simulink model "Quadrotor_Model_original"  (R2025b)
settings: Solver=ode45  StartTime=0.0  StopTime=15000  MaxStep=0.01  RelTol=1e-3  AbsTol=1e-4  EnableMultiTasking=on
values from neighbouring files (symbols this model uses):
  b = 0.07    [project_launch.m]
  g = 9.81    [project_launch.m]
  Jr = 1e-4    (= 0.0001)    [project_launch.m]
  k = 0.09    [project_launch.m]
  L = 0.225    [project_launch.m]
  m = 1.6    [project_launch.m]
libraries: slpidlib x5
settings Model: Creator=boyan  LastModifiedBy=neera
settings SolverCC: MaxConsecutiveMinStep=2  AlgebraicLoopSolver=TrustRegion
settings DataIOCC: LimitDataPoints=on  SaveFormat=Array  ReturnWorkspaceOutputs=off
settings OptimizationCC: LifeSpan=inf
settings DebuggingCC: SolverPrmCheckMsg=warning  UnconnectedInputMsg=warning  UnconnectedOutputMsg=warning  UnconnectedLineMsg=warning  SFUnexpectedBacktrackingDiag=warning  SFNoUnconditionalDefaultTransitionDiag=warning  SFExecutionAtInitializationDiag=none  ArithmeticOperatorsInVariantConditions=warning
settings HardwareCC: ProdBitPerPointer=32.0  ProdBitPerSizeT=32.0  ProdBitPerPtrDiffT=32.0  ProdLargestAtomicFloat=None  ProdIntDivRoundTo=Undefined  ProdEndianess=Unspecified  ProdWordSize=32.0  ProdHWDeviceType=32-bit Generic
settings ModelReferenceCC: EnableRefExpFcnMdlSchedulingChecks=on  PropagateSignalLabelsOutOfModel=off
settings SFSimCC: SimUseLocalCustomCode=off  CustomCodeUndefinedFunction=UseInterfaceOnly
settings RTWCC: RTWUseLocalCustomCode=off  GPUComputeCapability=3.5  DLArmComputeVersion=19.05
settings CodeAppCC: StateflowObjectComments=on
settings GRTTargetCC: TargetLangStandard=C89/C90 (ANSI)
settings ConfigComp: CovMetricSettings=dw  CovSaveCumulativeToWorkspaceVar=on  CovSaveSingleToWorkspaceVar=on  CovExternalEMLEnable=off  CovSFcnEnable=off

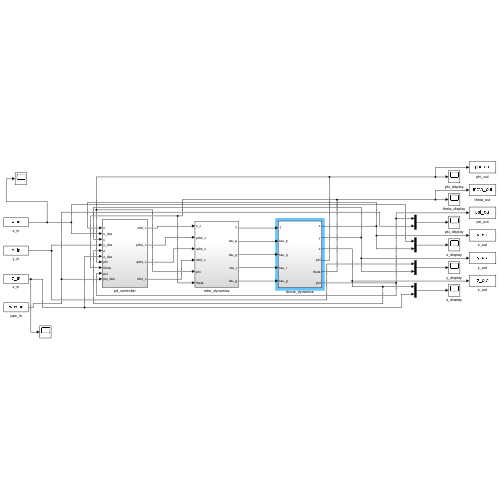
[thumbnail: Simulink's stored preview of the top-level diagram]
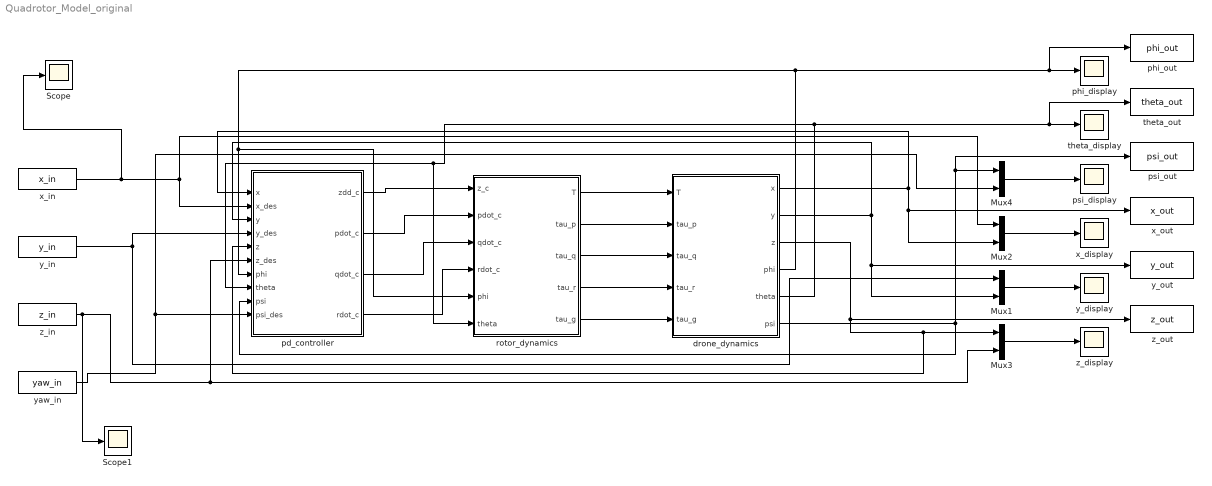
== system Quadrotor_Model_original ==
  Mux{1..4} (4 alike) : Mux  Inputs=2
  Scope : Scope
      settings: ActiveDisplayYMinimum=-3436.3102605592403  ActiveDisplayYMaximum=5145.090238480886  DataLoggingVariableName=ScopeData6
  Scope1 : Scope
      settings: ActiveDisplayYMinimum=-38.711321710722657  ActiveDisplayYMaximum=9.9150058205273481  DataLoggingVariableName=ScopeData7
  drone_dynamics : Subsystem
  pd_controller : Subsystem
  phi_display : Scope
      settings: ActiveDisplayYMinimum=-48.30659  ActiveDisplayYMaximum=31.01137
  phi_out : ToWorkspace  VariableName=phi_out  SaveFormat=Timeseries  SampleTime=-1
  psi_display : Scope
      settings: ActiveDisplayYMinimum=-104019.46579  ActiveDisplayYMaximum=26220.25866  DataLoggingVariableName=ScopeData2
  psi_out : ToWorkspace  VariableName=psi_out  SaveFormat=Timeseries  SampleTime=-1
  rotor_dynamics : Subsystem
  theta_display : Scope
      settings: ActiveDisplayYMinimum=-1.26378  ActiveDisplayYMaximum=0.84614  DataLoggingVariableName=ScopeData3
  theta_out : ToWorkspace  VariableName=theta_out  SaveFormat=Timeseries  SampleTime=-1
  x_display : Scope
      settings: ActiveDisplayYMinimum=-0.02581  ActiveDisplayYMaximum=0.17972  DataLoggingVariableName=ScopeData4
  x_in : FromWorkspace  VariableName=x_in
  x_out : ToWorkspace  VariableName=x_out  SaveFormat=Timeseries  SampleTime=-1
  y_display : Scope
      settings: ActiveDisplayYMinimum=98.09651  ActiveDisplayYMaximum=101.74643  DataLoggingVariableName=ScopeData5
  y_in : FromWorkspace  VariableName=y_in
  y_out : ToWorkspace  VariableName=y_out  SaveFormat=Timeseries  SampleTime=-1
  yaw_in : FromWorkspace  VariableName=yaw_in
  z_display : Scope
      settings: ActiveDisplayYMinimum=-47.57242  ActiveDisplayYMaximum=5.28582
  z_in : FromWorkspace  VariableName=z_in
  z_out : ToWorkspace  VariableName=z_out  SaveFormat=Timeseries  SampleTime=-1
  wires:
  rotor_dynamics/1(T) -> drone_dynamics/1(T)
  rotor_dynamics/2(tau_p) -> drone_dynamics/2(tau_p)
  pd_controller/1(zdd_c) -> rotor_dynamics/1(z_c)
  pd_controller/2(pdot_c) -> rotor_dynamics/2(pdot_c)
  z_in/1 -> pd_controller/6(z_des), Mux3/2, Scope1/1
  Mux1/1 -> y_display/1
  Mux2/1 -> x_display/1
  Mux4/1 -> psi_display/1
  Mux3/1 -> z_display/1
  drone_dynamics/6(psi) -> pd_controller/9(psi), psi_out/1, Mux4/1
  y_in/1 -> pd_controller/4(y_des), Mux1/1
  x_in/1 -> Scope/1, pd_controller/2(x_des), Mux2/1
  drone_dynamics/3(z) -> z_out/1, pd_controller/5(z), Mux3/1
  drone_dynamics/5(theta) -> theta_out/1, theta_display/1, pd_controller/8(theta), rotor_dynamics/6(theta)
  drone_dynamics/2(y) -> pd_controller/3(y), Mux1/2, y_out/1
  drone_dynamics/4(phi) -> phi_out/1, phi_display/1, pd_controller/7(phi), rotor_dynamics/5(phi)
  drone_dynamics/1(x) -> pd_controller/1(x), Mux2/2, x_out/1
  rotor_dynamics/5(tau_g) -> drone_dynamics/5(tau_g)
  rotor_dynamics/3(tau_q) -> drone_dynamics/3(tau_q)
  rotor_dynamics/4(tau_r) -> drone_dynamics/4(tau_r)
  yaw_in/1 -> pd_controller/10(psi_des), Mux4/2
  pd_controller/4(rdot_c) -> rotor_dynamics/4(rdot_c)
  pd_controller/3(qdot_c) -> rotor_dynamics/3(qdot_c)

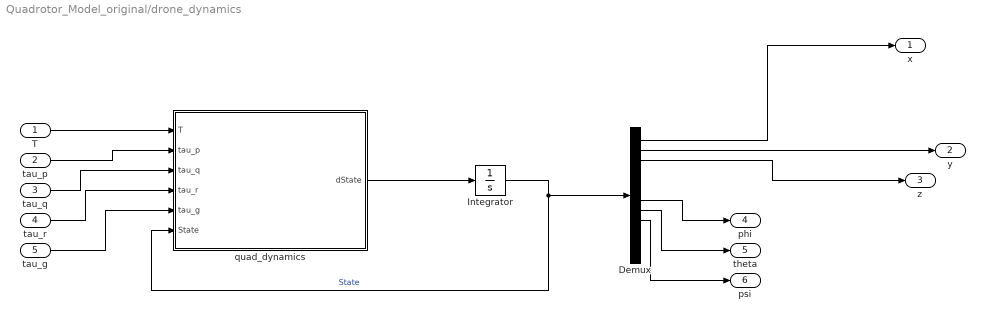
== system Quadrotor_Model_original/drone_dynamics ==
  T : Inport
  tau_p : Inport  Port=2
  tau_q : Inport  Port=3
  tau_r : Inport  Port=4
  tau_g : Inport  Port=5
  Demux : Demux  Outputs=12
  Integrator : Integrator  InitialCondition=[0; 0; 0; 0; 0; 0; 0; 0; 0; 0; 0; 0]
  quad_dynamics : MATLAB Function  TreatAsAtomicUnit=on
  x : Outport
  y : Outport  Port=2
  z : Outport  Port=3
  phi : Outport  Port=4
  theta : Outport  Port=5
  psi : Outport  Port=6
  wires:
  tau_p/1 -> quad_dynamics/2(tau_p)
  tau_q/1 -> quad_dynamics/3(tau_q)
  tau_r/1 -> quad_dynamics/4(tau_r)
  tau_g/1 -> quad_dynamics/5(tau_g)
  T/1 -> quad_dynamics/1(T)
  quad_dynamics/1(dState) -> Integrator/1
  Integrator/1 -> quad_dynamics/6(State), Demux/1  "State"
  Demux/7 -> phi/1
  Demux/8 -> theta/1
  Demux/9 -> psi/1
  Demux/1 -> x/1
  Demux/3 -> z/1
  Demux/2 -> y/1

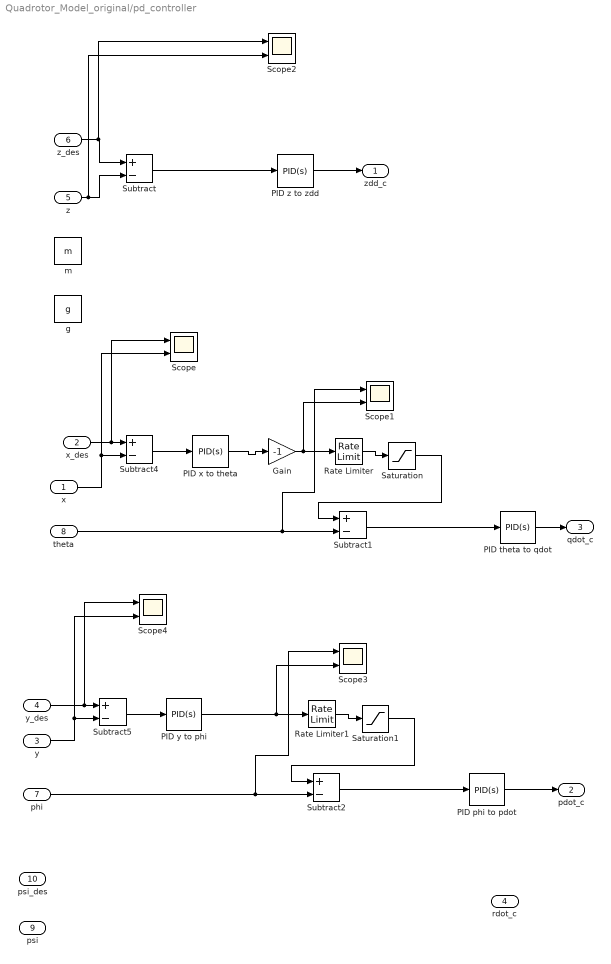
== system Quadrotor_Model_original/pd_controller ==
  x : Inport
  x_des : Inport  Port=2
  y : Inport  Port=3
  y_des : Inport  Port=4
  z : Inport  Port=5
  z_des : Inport  Port=6
  phi : Inport  Port=7
  theta : Inport  Port=8
  psi : Inport  Port=9
  psi_des : Inport  Port=10
  Gain : Gain  Gain=-1
  PID phi to pdot : slpidlib/PID Controller  Controller=PID  Form=Parallel  TimeDomain=Continuous-time  UseExternalTs=off  SampleTime=-1  IntegratorMethod=Forward Euler  FilterMethod=Forward Euler  ControllerParametersSource=internal  P=1  I=0  UseKiTs=off  D=0.5  UseExternalDerivativeSource=off  N=100  UseFilter=on  TunerSelectOption=Transfer Function Based (PID Tuner App)  InitialConditionSource=internal  InitialConditionForIntegrator=0  InitialConditionForFilter=0  DifferentiatorICPrevScaledInput=0  ExternalReset=none  TrackingMode=off  Kt=1  LimitOutput=off  SatLimitsSource=internal  UpperSaturationLimit=inf  LowerSaturationLimit=-inf  LinearizeAsGain=on  AntiWindupMode=none  Kb=1  LimitIntegrator=off  UpperIntegratorSaturationLimit=inf  LowerIntegratorSaturationLimit=-inf  POutMin=[]  POutMax=[]  IOutMin=[]  IOutMax=[]  DOutMin=[]  DOutMax=[]  NOutMin=[]  NOutMax=[]  SumOutMin=[]  SumOutMax=[]  SaturationOutMin=[]  SaturationOutMax=[]  PParamMin=[]  PParamMax=[]  IParamMin=[]  IParamMax=[]  DParamMin=[]  DParamMax=[]  NParamMin=[]  NParamMax=[]  KbParamMin=[]  KbParamMax=[]  KtParamMin=[]  KtParamMax=[]  KbOutMin=[]  KbOutMax=[]  KtOutMin=[]  KtOutMax=[]  IntegratorOutMin=[]  IntegratorOutMax=[]  FilterOutMin=[]  FilterOutMax=[]  SumI1OutMin=[]  SumI1OutMax=[]  SumI2OutMin=[]  SumI2OutMax=[]  SumI3OutMin=[]  SumI3OutMax=[]  SumI4OutMin=[]  SumI4OutMax=[]  SumDOutMin=[]  SumDOutMax=[]  DifferentiatorOutMin=[]  DifferentiatorOutMax=[]  FilterDiffOutCoefMin=[]  FilterDiffOutCoefMax=[]  ReciprocalOutMin=[]  ReciprocalOutMax=[]  SumDenOutMin=[]  SumDenOutMax=[]  SumNumOutMin=[]  SumNumOutMax=[]  DivideOutMin=[]  DivideOutMax=[]  UdiffTsProdOutMin=[]  UdiffTsProdOutMax=[]  NTsProdOutMin=[]  NTsProdOutMax=[]  UintegralTsProdOutMin=[]  UintegralTsProdOutMax=[]  UngainTsProdOutMin=[]  UngainTsProdOutMax=[]  ClampingZeroOutDataTypeStr=Inherit: Inherit via back propagation  ClampingZeroOutMin=[]  ClampingZeroOutMax=[]  FilterDenConstantOutDataTypeStr=Inherit: Inherit via back propagation  FilterDenConstantOutMin=[]  FilterDenConstantOutMax=[]  PCopyOutDataTypeStr=Inherit: Inherit via back propagation  PCopyOutMin=[]  PCopyOutMax=[]  NCopyOutDataTypeStr=Inherit: Inherit via back propagation  NCopyOutMin=[]  NCopyOutMax=[]  IntegratorContinuousStateAttributes=''  IntegratorStateMustResolveToSignalObject=off  IntegratorRTWStateStorageClass=Auto  FilterContinuousStateAttributes=''  FilterStateMustResolveToSignalObject=off  FilterRTWStateStorageClass=Auto  ParallelPVariant=InternalParameters  IdealPVariant=Disabled  IVariant=InternalParameters  DVariant=InternalParameters  IntegratorVariant=Continuous  SatVariant=Disabled  AWVariant=Passthrough  PCopyVariant=Disabled  TRVariant=Disabled  FdbkBlocksVariant=Forward  IdealPFdbkVariant=Disabled  SatFdbkVariant=Disabled  DerivativeFilterVariant=ContFilter  NVariant=InternalParameters  NCopyVariant=Disabled  FilterICVariant=InternalICsFilter  IntegratorICVariant=InternalICs  ExternalResetVariant=Disabled  TRSumVariant=Passthrough  SumFdbkVariant=Disabled  SumVariant=Sum_PID  TsampFilterVariant=InternalTs  TsampNgainVariant=Passthrough  TsampIntegralVariant=Disabled_SignalSpec  ExternalSaturationOutDataTypeStr=Inherit: Same as second input  DerivativeSourceVariant=ErrorSignal  PreIntVariant=InternalPreInt
  PID theta to qdot : slpidlib/PID Controller  Controller=PID  Form=Parallel  TimeDomain=Continuous-time  UseExternalTs=off  SampleTime=-1  IntegratorMethod=Forward Euler  FilterMethod=Forward Euler  ControllerParametersSource=internal  P=1  I=0  UseKiTs=off  D=0.5  UseExternalDerivativeSource=off  N=100  UseFilter=on  TunerSelectOption=Transfer Function Based (PID Tuner App)  InitialConditionSource=internal  InitialConditionForIntegrator=0  InitialConditionForFilter=0  DifferentiatorICPrevScaledInput=0  ExternalReset=none  TrackingMode=off  Kt=1  LimitOutput=off  SatLimitsSource=internal  UpperSaturationLimit=inf  LowerSaturationLimit=-inf  LinearizeAsGain=on  AntiWindupMode=none  Kb=1  LimitIntegrator=off  UpperIntegratorSaturationLimit=inf  LowerIntegratorSaturationLimit=-inf  POutMin=[]  POutMax=[]  IOutMin=[]  IOutMax=[]  DOutMin=[]  DOutMax=[]  NOutMin=[]  NOutMax=[]  SumOutMin=[]  SumOutMax=[]  SaturationOutMin=[]  SaturationOutMax=[]  PParamMin=[]  PParamMax=[]  IParamMin=[]  IParamMax=[]  DParamMin=[]  DParamMax=[]  NParamMin=[]  NParamMax=[]  KbParamMin=[]  KbParamMax=[]  KtParamMin=[]  KtParamMax=[]  KbOutMin=[]  KbOutMax=[]  KtOutMin=[]  KtOutMax=[]  IntegratorOutMin=[]  IntegratorOutMax=[]  FilterOutMin=[]  FilterOutMax=[]  SumI1OutMin=[]  SumI1OutMax=[]  SumI2OutMin=[]  SumI2OutMax=[]  SumI3OutMin=[]  SumI3OutMax=[]  SumI4OutMin=[]  SumI4OutMax=[]  SumDOutMin=[]  SumDOutMax=[]  DifferentiatorOutMin=[]  DifferentiatorOutMax=[]  FilterDiffOutCoefMin=[]  FilterDiffOutCoefMax=[]  ReciprocalOutMin=[]  ReciprocalOutMax=[]  SumDenOutMin=[]  SumDenOutMax=[]  SumNumOutMin=[]  SumNumOutMax=[]  DivideOutMin=[]  DivideOutMax=[]  UdiffTsProdOutMin=[]  UdiffTsProdOutMax=[]  NTsProdOutMin=[]  NTsProdOutMax=[]  UintegralTsProdOutMin=[]  UintegralTsProdOutMax=[]  UngainTsProdOutMin=[]  UngainTsProdOutMax=[]  ClampingZeroOutDataTypeStr=Inherit: Inherit via back propagation  ClampingZeroOutMin=[]  ClampingZeroOutMax=[]  FilterDenConstantOutDataTypeStr=Inherit: Inherit via back propagation  FilterDenConstantOutMin=[]  FilterDenConstantOutMax=[]  PCopyOutDataTypeStr=Inherit: Inherit via back propagation  PCopyOutMin=[]  PCopyOutMax=[]  NCopyOutDataTypeStr=Inherit: Inherit via back propagation  NCopyOutMin=[]  NCopyOutMax=[]  IntegratorContinuousStateAttributes=''  IntegratorStateMustResolveToSignalObject=off  IntegratorRTWStateStorageClass=Auto  FilterContinuousStateAttributes=''  FilterStateMustResolveToSignalObject=off  FilterRTWStateStorageClass=Auto  ParallelPVariant=InternalParameters  IdealPVariant=Disabled  IVariant=InternalParameters  DVariant=InternalParameters  IntegratorVariant=Continuous  SatVariant=Disabled  AWVariant=Passthrough  PCopyVariant=Disabled  TRVariant=Disabled  FdbkBlocksVariant=Forward  IdealPFdbkVariant=Disabled  SatFdbkVariant=Disabled  DerivativeFilterVariant=ContFilter  NVariant=InternalParameters  NCopyVariant=Disabled  FilterICVariant=InternalICsFilter  IntegratorICVariant=InternalICs  ExternalResetVariant=Disabled  TRSumVariant=Passthrough  SumFdbkVariant=Disabled  SumVariant=Sum_PID  TsampFilterVariant=InternalTs  TsampNgainVariant=Passthrough  TsampIntegralVariant=Disabled_SignalSpec  ExternalSaturationOutDataTypeStr=Inherit: Same as second input  DerivativeSourceVariant=ErrorSignal  PreIntVariant=InternalPreInt
  PID x to theta : slpidlib/PID Controller  Controller=PID  Form=Parallel  TimeDomain=Continuous-time  UseExternalTs=off  SampleTime=-1  IntegratorMethod=Forward Euler  FilterMethod=Forward Euler  ControllerParametersSource=internal  P=0.004  I=0  UseKiTs=off  D=0.0003  UseExternalDerivativeSource=off  N=100  UseFilter=on  TunerSelectOption=Transfer Function Based (PID Tuner App)  InitialConditionSource=internal  InitialConditionForIntegrator=0  InitialConditionForFilter=0  DifferentiatorICPrevScaledInput=0  ExternalReset=none  TrackingMode=off  Kt=1  LimitOutput=off  SatLimitsSource=internal  UpperSaturationLimit=inf  LowerSaturationLimit=-inf  LinearizeAsGain=on  AntiWindupMode=none  Kb=1  LimitIntegrator=off  UpperIntegratorSaturationLimit=inf  LowerIntegratorSaturationLimit=-inf  POutMin=[]  POutMax=[]  IOutMin=[]  IOutMax=[]  DOutMin=[]  DOutMax=[]  NOutMin=[]  NOutMax=[]  SumOutMin=[]  SumOutMax=[]  SaturationOutMin=[]  SaturationOutMax=[]  PParamMin=[]  PParamMax=[]  IParamMin=[]  IParamMax=[]  DParamMin=[]  DParamMax=[]  NParamMin=[]  NParamMax=[]  KbParamMin=[]  KbParamMax=[]  KtParamMin=[]  KtParamMax=[]  KbOutMin=[]  KbOutMax=[]  KtOutMin=[]  KtOutMax=[]  IntegratorOutMin=[]  IntegratorOutMax=[]  FilterOutMin=[]  FilterOutMax=[]  SumI1OutMin=[]  SumI1OutMax=[]  SumI2OutMin=[]  SumI2OutMax=[]  SumI3OutMin=[]  SumI3OutMax=[]  SumI4OutMin=[]  SumI4OutMax=[]  SumDOutMin=[]  SumDOutMax=[]  DifferentiatorOutMin=[]  DifferentiatorOutMax=[]  FilterDiffOutCoefMin=[]  FilterDiffOutCoefMax=[]  ReciprocalOutMin=[]  ReciprocalOutMax=[]  SumDenOutMin=[]  SumDenOutMax=[]  SumNumOutMin=[]  SumNumOutMax=[]  DivideOutMin=[]  DivideOutMax=[]  UdiffTsProdOutMin=[]  UdiffTsProdOutMax=[]  NTsProdOutMin=[]  NTsProdOutMax=[]  UintegralTsProdOutMin=[]  UintegralTsProdOutMax=[]  UngainTsProdOutMin=[]  UngainTsProdOutMax=[]  ClampingZeroOutDataTypeStr=Inherit: Inherit via back propagation  ClampingZeroOutMin=[]  ClampingZeroOutMax=[]  FilterDenConstantOutDataTypeStr=Inherit: Inherit via back propagation  FilterDenConstantOutMin=[]  FilterDenConstantOutMax=[]  PCopyOutDataTypeStr=Inherit: Inherit via back propagation  PCopyOutMin=[]  PCopyOutMax=[]  NCopyOutDataTypeStr=Inherit: Inherit via back propagation  NCopyOutMin=[]  NCopyOutMax=[]  IntegratorContinuousStateAttributes=''  IntegratorStateMustResolveToSignalObject=off  IntegratorRTWStateStorageClass=Auto  FilterContinuousStateAttributes=''  FilterStateMustResolveToSignalObject=off  FilterRTWStateStorageClass=Auto  ParallelPVariant=InternalParameters  IdealPVariant=Disabled  IVariant=InternalParameters  DVariant=InternalParameters  IntegratorVariant=Continuous  SatVariant=Disabled  AWVariant=Passthrough  PCopyVariant=Disabled  TRVariant=Disabled  FdbkBlocksVariant=Forward  IdealPFdbkVariant=Disabled  SatFdbkVariant=Disabled  DerivativeFilterVariant=ContFilter  NVariant=InternalParameters  NCopyVariant=Disabled  FilterICVariant=InternalICsFilter  IntegratorICVariant=InternalICs  ExternalResetVariant=Disabled  TRSumVariant=Passthrough  SumFdbkVariant=Disabled  SumVariant=Sum_PID  TsampFilterVariant=InternalTs  TsampNgainVariant=Passthrough  TsampIntegralVariant=Disabled_SignalSpec  ExternalSaturationOutDataTypeStr=Inherit: Same as second input  DerivativeSourceVariant=ErrorSignal  PreIntVariant=InternalPreInt
  PID y to phi : slpidlib/PID Controller  Controller=PID  Form=Parallel  TimeDomain=Continuous-time  UseExternalTs=off  SampleTime=-1  IntegratorMethod=Forward Euler  FilterMethod=Forward Euler  ControllerParametersSource=internal  P=0.003  I=0  UseKiTs=off  D=0.0001  UseExternalDerivativeSource=off  N=100  UseFilter=on  TunerSelectOption=Transfer Function Based (PID Tuner App)  InitialConditionSource=internal  InitialConditionForIntegrator=0  InitialConditionForFilter=0  DifferentiatorICPrevScaledInput=0  ExternalReset=none  TrackingMode=off  Kt=1  LimitOutput=off  SatLimitsSource=internal  UpperSaturationLimit=inf  LowerSaturationLimit=-inf  LinearizeAsGain=on  AntiWindupMode=none  Kb=1  LimitIntegrator=off  UpperIntegratorSaturationLimit=inf  LowerIntegratorSaturationLimit=-inf  POutMin=[]  POutMax=[]  IOutMin=[]  IOutMax=[]  DOutMin=[]  DOutMax=[]  NOutMin=[]  NOutMax=[]  SumOutMin=[]  SumOutMax=[]  SaturationOutMin=[]  SaturationOutMax=[]  PParamMin=[]  PParamMax=[]  IParamMin=[]  IParamMax=[]  DParamMin=[]  DParamMax=[]  NParamMin=[]  NParamMax=[]  KbParamMin=[]  KbParamMax=[]  KtParamMin=[]  KtParamMax=[]  KbOutMin=[]  KbOutMax=[]  KtOutMin=[]  KtOutMax=[]  IntegratorOutMin=[]  IntegratorOutMax=[]  FilterOutMin=[]  FilterOutMax=[]  SumI1OutMin=[]  SumI1OutMax=[]  SumI2OutMin=[]  SumI2OutMax=[]  SumI3OutMin=[]  SumI3OutMax=[]  SumI4OutMin=[]  SumI4OutMax=[]  SumDOutMin=[]  SumDOutMax=[]  DifferentiatorOutMin=[]  DifferentiatorOutMax=[]  FilterDiffOutCoefMin=[]  FilterDiffOutCoefMax=[]  ReciprocalOutMin=[]  ReciprocalOutMax=[]  SumDenOutMin=[]  SumDenOutMax=[]  SumNumOutMin=[]  SumNumOutMax=[]  DivideOutMin=[]  DivideOutMax=[]  UdiffTsProdOutMin=[]  UdiffTsProdOutMax=[]  NTsProdOutMin=[]  NTsProdOutMax=[]  UintegralTsProdOutMin=[]  UintegralTsProdOutMax=[]  UngainTsProdOutMin=[]  UngainTsProdOutMax=[]  ClampingZeroOutDataTypeStr=Inherit: Inherit via back propagation  ClampingZeroOutMin=[]  ClampingZeroOutMax=[]  FilterDenConstantOutDataTypeStr=Inherit: Inherit via back propagation  FilterDenConstantOutMin=[]  FilterDenConstantOutMax=[]  PCopyOutDataTypeStr=Inherit: Inherit via back propagation  PCopyOutMin=[]  PCopyOutMax=[]  NCopyOutDataTypeStr=Inherit: Inherit via back propagation  NCopyOutMin=[]  NCopyOutMax=[]  IntegratorContinuousStateAttributes=''  IntegratorStateMustResolveToSignalObject=off  IntegratorRTWStateStorageClass=Auto  FilterContinuousStateAttributes=''  FilterStateMustResolveToSignalObject=off  FilterRTWStateStorageClass=Auto  ParallelPVariant=InternalParameters  IdealPVariant=Disabled  IVariant=InternalParameters  DVariant=InternalParameters  IntegratorVariant=Continuous  SatVariant=Disabled  AWVariant=Passthrough  PCopyVariant=Disabled  TRVariant=Disabled  FdbkBlocksVariant=Forward  IdealPFdbkVariant=Disabled  SatFdbkVariant=Disabled  DerivativeFilterVariant=ContFilter  NVariant=InternalParameters  NCopyVariant=Disabled  FilterICVariant=InternalICsFilter  IntegratorICVariant=InternalICs  ExternalResetVariant=Disabled  TRSumVariant=Passthrough  SumFdbkVariant=Disabled  SumVariant=Sum_PID  TsampFilterVariant=InternalTs  TsampNgainVariant=Passthrough  TsampIntegralVariant=Disabled_SignalSpec  ExternalSaturationOutDataTypeStr=Inherit: Same as second input  DerivativeSourceVariant=ErrorSignal  PreIntVariant=InternalPreInt
  PID z to zdd : slpidlib/PID Controller  Controller=PID  Form=Parallel  TimeDomain=Continuous-time  UseExternalTs=off  SampleTime=-1  IntegratorMethod=Forward Euler  FilterMethod=Forward Euler  ControllerParametersSource=internal  P=0.15  I=0  UseKiTs=off  D=1  UseExternalDerivativeSource=off  N=100  UseFilter=on  TunerSelectOption=Transfer Function Based (PID Tuner App)  InitialConditionSource=internal  InitialConditionForIntegrator=0  InitialConditionForFilter=0  DifferentiatorICPrevScaledInput=0  ExternalReset=none  TrackingMode=off  Kt=1  LimitOutput=off  SatLimitsSource=internal  UpperSaturationLimit=inf  LowerSaturationLimit=-inf  LinearizeAsGain=on  AntiWindupMode=none  Kb=1  LimitIntegrator=off  UpperIntegratorSaturationLimit=inf  LowerIntegratorSaturationLimit=-inf  POutMin=[]  POutMax=[]  IOutMin=[]  IOutMax=[]  DOutMin=[]  DOutMax=[]  NOutMin=[]  NOutMax=[]  SumOutMin=[]  SumOutMax=[]  SaturationOutMin=[]  SaturationOutMax=[]  PParamMin=[]  PParamMax=[]  IParamMin=[]  IParamMax=[]  DParamMin=[]  DParamMax=[]  NParamMin=[]  NParamMax=[]  KbParamMin=[]  KbParamMax=[]  KtParamMin=[]  KtParamMax=[]  KbOutMin=[]  KbOutMax=[]  KtOutMin=[]  KtOutMax=[]  IntegratorOutMin=[]  IntegratorOutMax=[]  FilterOutMin=[]  FilterOutMax=[]  SumI1OutMin=[]  SumI1OutMax=[]  SumI2OutMin=[]  SumI2OutMax=[]  SumI3OutMin=[]  SumI3OutMax=[]  SumI4OutMin=[]  SumI4OutMax=[]  SumDOutMin=[]  SumDOutMax=[]  DifferentiatorOutMin=[]  DifferentiatorOutMax=[]  FilterDiffOutCoefMin=[]  FilterDiffOutCoefMax=[]  ReciprocalOutMin=[]  ReciprocalOutMax=[]  SumDenOutMin=[]  SumDenOutMax=[]  SumNumOutMin=[]  SumNumOutMax=[]  DivideOutMin=[]  DivideOutMax=[]  UdiffTsProdOutMin=[]  UdiffTsProdOutMax=[]  NTsProdOutMin=[]  NTsProdOutMax=[]  UintegralTsProdOutMin=[]  UintegralTsProdOutMax=[]  UngainTsProdOutMin=[]  UngainTsProdOutMax=[]  ClampingZeroOutDataTypeStr=Inherit: Inherit via back propagation  ClampingZeroOutMin=[]  ClampingZeroOutMax=[]  FilterDenConstantOutDataTypeStr=Inherit: Inherit via back propagation  FilterDenConstantOutMin=[]  FilterDenConstantOutMax=[]  PCopyOutDataTypeStr=Inherit: Inherit via back propagation  PCopyOutMin=[]  PCopyOutMax=[]  NCopyOutDataTypeStr=Inherit: Inherit via back propagation  NCopyOutMin=[]  NCopyOutMax=[]  IntegratorContinuousStateAttributes=''  IntegratorStateMustResolveToSignalObject=off  IntegratorRTWStateStorageClass=Auto  FilterContinuousStateAttributes=''  FilterStateMustResolveToSignalObject=off  FilterRTWStateStorageClass=Auto  ParallelPVariant=InternalParameters  IdealPVariant=Disabled  IVariant=InternalParameters  DVariant=InternalParameters  IntegratorVariant=Continuous  SatVariant=Disabled  AWVariant=Passthrough  PCopyVariant=Disabled  TRVariant=Disabled  FdbkBlocksVariant=Forward  IdealPFdbkVariant=Disabled  SatFdbkVariant=Disabled  DerivativeFilterVariant=ContFilter  NVariant=InternalParameters  NCopyVariant=Disabled  FilterICVariant=InternalICsFilter  IntegratorICVariant=InternalICs  ExternalResetVariant=Disabled  TRSumVariant=Passthrough  SumFdbkVariant=Disabled  SumVariant=Sum_PID  TsampFilterVariant=InternalTs  TsampNgainVariant=Passthrough  TsampIntegralVariant=Disabled_SignalSpec  ExternalSaturationOutDataTypeStr=Inherit: Same as second input  DerivativeSourceVariant=ErrorSignal  PreIntVariant=InternalPreInt
  Rate Limiter : RateLimiter  RisingSlewLimit=0.3  FallingSlewLimit=-0.3  SampleTimeMode=inherited
  Rate Limiter1 : RateLimiter  RisingSlewLimit=0.3  FallingSlewLimit=-0.3  SampleTimeMode=inherited
  Saturation : Saturate  UpperLimit=0.2  LowerLimit=-0.2
  Saturation1 : Saturate  UpperLimit=0.2  LowerLimit=-0.2
  Scope{,1..4} (5 alike) : Scope  NumInputPorts=2
      Scope settings: ActiveDisplayYMinimum=-98.733416705129031  ActiveDisplayYMaximum=43.1887874753256  DataLoggingVariableName=ScopeData8
      Scope1 settings: ActiveDisplayYMinimum=-0.5554469417713892  ActiveDisplayYMaximum=0.80861740055255715  DataLoggingVariableName=ScopeData10
      Scope2 settings: ActiveDisplayYMinimum=-30.514783869107124  ActiveDisplayYMaximum=-30.145005447762422  DataLoggingVariableName=ScopeData11
      Scope3 settings: ActiveDisplayYMinimum=-0.5554469417713892  ActiveDisplayYMaximum=0.80861740055255715  DataLoggingVariableName=ScopeData12
      Scope4 settings: ActiveDisplayYMinimum=-4980.6193239584863  ActiveDisplayYMaximum=553.40214710649832  DataLoggingVariableName=ScopeData13
  Subtract{,1..2,4..5} (5 alike) : Sum  Inputs=+-
  g : Constant  Value=g
  m : Constant  Value=m
  zdd_c : Outport
  pdot_c : Outport  Port=2
  qdot_c : Outport  Port=3
  rdot_c : Outport  Port=4
  wires:
  z_des/1 -> Scope2/1, Subtract/1
  z/1 -> Scope2/2, Subtract/2
  Subtract/1 -> PID z to zdd/1
  theta/1 -> Scope1/1, Subtract1/2
  x/1 -> Scope/2, Subtract4/2
  Subtract4/1 -> PID x to theta/1
  PID x to theta/1 -> Gain/1
  Subtract1/1 -> PID theta to qdot/1
  Saturation/1 -> Subtract1/1
  Gain/1 -> Rate Limiter/1, Scope1/2
  x_des/1 -> Scope/1, Subtract4/1
  Rate Limiter/1 -> Saturation/1
  Rate Limiter1/1 -> Saturation1/1
  y/1 -> Scope4/2, Subtract5/2
  y_des/1 -> Scope4/1, Subtract5/1
  phi/1 -> Scope3/1, Subtract2/2
  PID y to phi/1 -> Rate Limiter1/1, Scope3/2
  Subtract5/1 -> PID y to phi/1
  Subtract2/1 -> PID phi to pdot/1
  Saturation1/1 -> Subtract2/1
  PID phi to pdot/1 -> pdot_c/1
  PID theta to qdot/1 -> qdot_c/1
  PID z to zdd/1 -> zdd_c/1

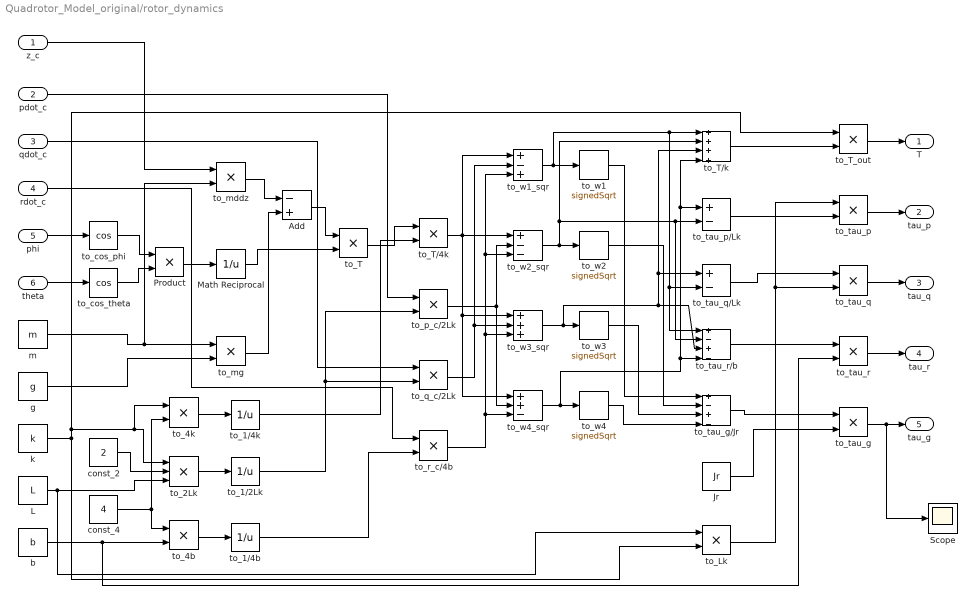
== system Quadrotor_Model_original/rotor_dynamics ==
  z_c : Inport
  pdot_c : Inport  Port=2
  qdot_c : Inport  Port=3
  rdot_c : Inport  Port=4
  phi : Inport  Port=5
  theta : Inport  Port=6
  Add : Sum  Inputs=-+
  Jr : Constant  Value=Jr
  L : Constant  Value=L
  Math Reciprocal : Math  Operator=reciprocal  SignedPower=on
  Product : Product
  Scope : Scope
      settings: ActiveDisplayYMinimum=-1  ActiveDisplayYMaximum=1  DataLoggingVariableName=ScopeData9
  b : Constant  Value=b
  const_2 : Constant  Value=2
  const_4 : Constant  Value=4
  g : Constant  Value=g
  k : Constant  Value=k
  m : Constant  Value=m
  to_1/2Lk : Math  Operator=reciprocal  SignedPower=on
  to_1/4b : Math  Operator=reciprocal  SignedPower=on
  to_1/4k : Math  Operator=reciprocal  SignedPower=on
  to_2Lk : Product  Inputs=3
  to_4b : Product
  to_4k : Product
  to_Lk : Product
  to_T : Product
  to_T/4k : Product
  to_T/k : Sum  Inputs=++++
  to_T_out : Product
  to_cos_phi : Trigonometry  Operator=cos
  to_cos_theta : Trigonometry  Operator=cos
  to_mddz : Product
  to_mg : Product
  to_p_c/2Lk : Product
  to_q_c/2Lk : Product
  to_r_c/4b : Product
  to_tau_g : Product
  to_tau_g/Jr : Sum  Inputs=+-+-
  to_tau_p : Product
  to_tau_p/Lk : Sum  Inputs=+-
  to_tau_q : Product
  to_tau_q/Lk : Sum  Inputs=+-
  to_tau_r : Product
  to_tau_r/b : Sum  Inputs=+-+-
  to_w{1..4} (4 alike) : Sqrt  Operator=signedSqrt
  to_w1_sqr : Sum  Inputs=+-+
  to_w2_sqr : Sum  Inputs=+--
  to_w3_sqr : Sum  Inputs=+++
  to_w4_sqr : Sum  Inputs=++-
  T : Outport
  tau_p : Outport  Port=2
  tau_q : Outport  Port=3
  tau_r : Outport  Port=4
  tau_g : Outport  Port=5
  wires:
  phi/1 -> to_cos_phi/1
  theta/1 -> to_cos_theta/1
  to_cos_phi/1 -> Product/1
  to_cos_theta/1 -> Product/2
  Product/1 -> Math Reciprocal/1
  m/1 -> to_mddz/2, to_mg/1
  g/1 -> to_mg/2
  to_mg/1 -> Add/2
  Math Reciprocal/1 -> to_T/2
  Add/1 -> to_T/1
  k/1 -> to_2Lk/1, to_4k/1, to_T_out/1, to_Lk/2
  const_4/1 -> to_4b/1, to_4k/2
  const_2/1 -> to_2Lk/2
  L/1 -> to_2Lk/3, to_Lk/1
  b/1 -> to_tau_r/2, to_4b/2
  to_4k/1 -> to_1/4k/1
  to_2Lk/1 -> to_1/2Lk/1
  to_4b/1 -> to_1/4b/1
  to_T/1 -> to_T/4k/1
  to_1/4k/1 -> to_T/4k/2
  pdot_c/1 -> to_p_c/2Lk/1
  to_1/2Lk/1 -> to_q_c/2Lk/2, to_p_c/2Lk/2
  qdot_c/1 -> to_q_c/2Lk/1
  to_1/4b/1 -> to_r_c/4b/2
  rdot_c/1 -> to_r_c/4b/1
  to_T/4k/1 -> to_w2_sqr/1, to_w3_sqr/1, to_w4_sqr/1, to_w1_sqr/1
  to_q_c/2Lk/1 -> to_w3_sqr/2, to_w1_sqr/2
  to_r_c/4b/1 -> to_w4_sqr/3, to_w3_sqr/3, to_w2_sqr/3, to_w1_sqr/3
  to_p_c/2Lk/1 -> to_w2_sqr/2, to_w4_sqr/2
  to_w1_sqr/1 -> to_w1/1, to_tau_r/b/1, to_tau_q/Lk/2, to_T/k/1
  to_w2_sqr/1 -> to_w2/1, to_tau_r/b/2, to_tau_p/Lk/2, to_T/k/2
  to_w3_sqr/1 -> to_w3/1, to_tau_q/Lk/1, to_T/k/3, to_tau_r/b/3
  to_w4_sqr/1 -> to_w4/1, to_tau_p/Lk/1, to_T/k/4, to_tau_r/b/4
  to_w2/1 -> to_tau_g/Jr/2
  to_w1/1 -> to_tau_g/Jr/1
  to_w3/1 -> to_tau_g/Jr/3
  to_w4/1 -> to_tau_g/Jr/4
  to_T_out/1 -> T/1
  to_T/k/1 -> to_T_out/2
  to_tau_p/1 -> tau_p/1
  to_tau_p/Lk/1 -> to_tau_p/2
  to_tau_q/1 -> tau_q/1
  to_tau_r/1 -> tau_r/1
  to_tau_r/b/1 -> to_tau_r/1
  to_tau_q/Lk/1 -> to_tau_q/1
  to_tau_g/1 -> Scope/1, tau_g/1
  to_Lk/1 -> to_tau_p/1, to_tau_q/2
  Jr/1 -> to_tau_g/2
  z_c/1 -> to_mddz/1
  to_mddz/1 -> Add/1
  to_tau_g/Jr/1 -> to_tau_g/1

== matlab function Quadrotor_Model_original/drone_dynamics/quad_dynamics ==
  data: T input; dState output size=12; tau_p input; tau_q input; tau_r input; tau_g input; State input
function dState = fcn(T, tau_p, tau_q, tau_r, tau_g, State)
    % Parameters
    m   = 1.6;
    g   = 9.81;
    Ixx = 0.03;
    Iyy = 0.03;
    Izz = 0.06;

    % Unpack state
    x_dot = State(4);
    y_dot = State(5);
    z_dot = State(6);
    phi   = State(7);
    theta = State(8);
    psi   = State(9);
    p     = State(10);
    q     = State(11);
    r     = State(12);

    % ---------- PHYSICAL LIMITS (CRITICAL) ----------
    % Thrust: [0, 3g]
    T_hover = m * g;
    T = max(0, min(3*T_hover, T));

    % Torques: [-3, 3] N·m
    tau_max = 3;
    tau_p = max(-tau_max, min(tau_max, tau_p));
    tau_q = max(-tau_max, min(tau_max, tau_q));
    tau_r = max(-tau_max, min(tau_max, tau_r));

    % Also limit angular rates a bit
    w_max = 50;       % rad/s
    p = max(-w_max, min(w_max, p));
    q = max(-w_max, min(w_max, q));
    r = max(-w_max, min(w_max, r));
    % ------------------------------------------------

    % Trig
    cphi = cos(phi);  sphi = sin(phi);
    cthe = cos(theta); sthe = sin(theta);
    cpsi = cos(psi);  spsi = sin(psi);

    % protect cos(theta)
    eps_cos = 1e-3;
    if abs(cthe) < eps_cos
        cthe = eps_cos * sign(cthe + (cthe==0));
    end

    % Translational dynamics (NED)
    x_dd = -(T/m) * (cphi*sthe*cpsi + sphi*spsi);
    y_dd = -(T/m) * (cphi*sthe*spsi - sphi*cpsi);
    z_dd =  g     - (T/m) * (cphi*cthe);

    % Gyro torques
    tau_gx = -tau_g * q;
    tau_gy =  tau_g * p;
    tau_gz =  0;

    p_dot = (tau_p + tau_gx + (Iyy - Izz)*q*r) / Ixx;
    q_dot = (tau_q + tau_gy + (Izz - Ixx)*p*r) / Iyy;
    r_dot = (tau_r + tau_gz + (Ixx - Iyy)*p*q) / Izz;

    % Euler kinematics
    tt = sthe / cthe;
    phi_dot   = p + (q*sphi + r*cphi) * tt;
    theta_dot = q*cphi - r*sphi;
    psi_dot   = (q*sphi + r*cphi) / cthe;

    % Pack
    dState = [ ...
        x_dot; y_dot; z_dot; ...
        x_dd;  y_dd;  z_dd;  ...
        phi_dot; theta_dot; psi_dot; ...
        p_dot; q_dot; r_dot ...
    ];
end
